simulink model "mpc_bike_model"  (R2018b)
settings: Solver=ode23s  StartTime=0.0  StopTime=sim_time  FixedStep=Ts_IMU  MaxStep=Ts  RelTol=1e-3
values from neighbouring files (symbols this model uses):
  A_kalman = [1 0 Ts 0; 0 1 0 Ts; 0 0 1 0; 0 0 0 1]    [configuration_boxMovedCenter.m]    (also in configuration_lqrTuning.m; configuration_pidTuning.m; configuration_yixiao.m)
  b_compFilter = b_real    (= 1.095)    [configuration_boxMovedCenter.m]    (also in configuration_lqrTuning.m; configuration_pidTuning.m; configuration_yixiao.m)
  B_kalman = [0 0 0 0; 0 0 0 0; 0 0 0 0; 0 0 0 0]    [configuration_boxMovedCenter.m]    (also in configuration_lqrTuning.m; configuration_pidTuning.m; configuration_yixiao.m)
  b_real = 1.095    [configuration_boxMovedCenter.m]    (also in configuration_lqrTuning.m; configuration_pidTuning.m; configuration_yixiao.m)
  C_kalman = [1 0 0 0; 0 1 0 0; 0 0 1 0; 0 0 0 1]    [configuration_boxMovedCenter.m]    (also in configuration_lqrTuning.m; configuration_pidTuning.m; configuration_yixiao.m)
  complementary = 0.985    [configuration_boxMovedCenter.m]    (also in configuration_lqrTuning.m; configuration_pidTuning.m; configuration_yixiao.m)
  D_kalman = [0 0 0 0; 0 0 0 0; 0 0 0 0; 0 0 0 0]    [configuration_boxMovedCenter.m]    (also in configuration_lqrTuning.m; configuration_pidTuning.m; configuration_yixiao.m)
  damp = 0.4    [configuration_boxMovedCenter.m]    (also in configuration_lqrTuning.m; configuration_pidTuning.m; configuration_yixiao.m)
  Dead_Band = [0.0, -0.0, 0.0]    [configuration_boxMovedCenter.m]    (also in configuration_lqrTuning.m = [0.055, -0.055, 0.005]; configuration_pidTuning.m = [0.055, -0.055, 0.005]; configuration_yixiao.m = [0.055, -0.055, 0.005])
  delay = 0.045    [configuration_boxMovedCenter.m]    (also in configuration_lqrTuning.m; configuration_pidTuning.m; configuration_yixiao.m)
  direct_control = 1    [configuration_boxMovedCenter.m]    (also in configuration_lqrTuning.m; configuration_pidTuning.m; configuration_yixiao.m)
  filter_model = 1    [configuration_boxMovedCenter.m]    (also in configuration_lqrTuning.m; configuration_pidTuning.m; configuration_yixiao.m)
  forward_motor_dynamics = 0    [configuration_boxMovedCenter.m]    (also in configuration_lqrTuning.m; configuration_pidTuning.m; configuration_yixiao.m)
  fr_oscil = 1    [configuration_boxMovedCenter.m]    (also in configuration_lqrTuning.m; configuration_pidTuning.m; configuration_yixiao.m)
  g = 9.81    [configuration_boxMovedCenter.m]    (also in configuration_lqrTuning.m; configuration_pidTuning.m; configuration_yixiao.m)
  gain = 0.3    [configuration_boxMovedCenter.m]    (also in configuration_lqrTuning.m; configuration_pidTuning.m; configuration_yixiao.m)
  I_direct = 0.4    [configuration_boxMovedCenter.m]    (also in configuration_lqrTuning.m = 0.000227125326188; configuration_pidTuning.m = 0.000227125326188; configuration_yixiao.m)
  I_lat = 0.01    [configuration_boxMovedCenter.m]    (also in configuration_lqrTuning.m = 0.000115580509654; configuration_pidTuning.m = 0.000115580509654; configuration_yixiao.m)
  I_steer = 0.1    [configuration_boxMovedCenter.m]    (also in configuration_lqrTuning.m = 0.451012019539; configuration_pidTuning.m = 0.451012019539; configuration_yixiao.m = 0.3)
  IMU_height_model = 0.45    [configuration_boxMovedCenter.m]    (also in configuration_lqrTuning.m; configuration_pidTuning.m; configuration_yixiao.m)
  IMU_height_real = 0.45    [configuration_boxMovedCenter.m]    (also in configuration_lqrTuning.m; configuration_pidTuning.m; configuration_yixiao.m)
  initial_states = [deg2rad(5) deg2rad(-2) deg2rad(0)]    [configuration_boxMovedCenter.m]    (also in configuration_lqrTuning.m = [deg2rad(-2) deg2rad(0) deg2rad(0)]; configuration_pidTuning.m = [deg2rad(-2) deg2rad(0) deg2rad(0)]; configuration_yixiao.m = [deg2rad(-2) deg2rad(0) deg2rad(0)])
  input_velocity = 3    [configuration_boxMovedCenter.m]    (also in configuration_lqrTuning.m; configuration_pidTuning.m; configuration_yixiao.m)
  lambda_compFilter = deg2rad(70)    [configuration_boxMovedCenter.m]    (also in configuration_lqrTuning.m; configuration_pidTuning.m; configuration_yixiao.m)
  lambda_real = deg2rad(70)    [configuration_boxMovedCenter.m]    (also in configuration_lqrTuning.m; configuration_pidTuning.m; configuration_yixiao.m)
  lat_control = 1    [configuration_boxMovedCenter.m]    (also in configuration_lqrTuning.m; configuration_pidTuning.m; configuration_yixiao.m)
  look_ahead = 0    [configuration_boxMovedCenter.m]    (also in configuration_lqrTuning.m; configuration_pidTuning.m; configuration_yixiao.m)
  max_handlebar = 40*(pi/180)    (= 0.698131700798)    [configuration_boxMovedCenter.m]    (also in configuration_lqrTuning.m; configuration_pidTuning.m; configuration_yixiao.m)
  max_roll = pi/2    (= 1.57079632679)    [configuration_boxMovedCenter.m]    (also in configuration_lqrTuning.m; configuration_pidTuning.m; configuration_yixiao.m)
  max_steering_motor_acc = inf    [configuration_boxMovedCenter.m]    (also in configuration_lqrTuning.m; configuration_pidTuning.m; configuration_yixiao.m)
  max_steering_motor_speed = 7.5    [configuration_boxMovedCenter.m]    (also in configuration_lqrTuning.m; configuration_pidTuning.m; configuration_yixiao.m)
  min_handlebar = -max_handlebar    (= -0.698131700798)    [configuration_boxMovedCenter.m]    (also in configuration_lqrTuning.m; configuration_pidTuning.m; configuration_yixiao.m)
  min_roll = - max_roll    (= -1.57079632679)    [configuration_boxMovedCenter.m]    (also in configuration_lqrTuning.m; configuration_pidTuning.m; configuration_yixiao.m)
  min_steering_motor_acc = -inf    [configuration_boxMovedCenter.m]    (also in configuration_lqrTuning.m; configuration_pidTuning.m; configuration_yixiao.m)
  min_steering_motor_speed = -7.5    [configuration_boxMovedCenter.m]    (also in configuration_lqrTuning.m; configuration_pidTuning.m; configuration_yixiao.m)
  noise = 1    [configuration_boxMovedCenter.m]    (also in configuration_lqrTuning.m = 0; configuration_pidTuning.m = 0; configuration_yixiao.m = 0)
  noise_acc = 2.4869e-05    [configuration_boxMovedCenter.m]    (also in configuration_lqrTuning.m; configuration_pidTuning.m; configuration_yixiao.m)
  noise_encoder = 1e-7    (= 1e-07)    [configuration_boxMovedCenter.m]    (also in configuration_lqrTuning.m; configuration_pidTuning.m; configuration_yixiao.m)
  noise_gyro = 0.0022    [configuration_boxMovedCenter.m]    (also in configuration_lqrTuning.m; configuration_pidTuning.m; configuration_yixiao.m)
  noise_hall = 0.0031    [configuration_boxMovedCenter.m]    (also in configuration_lqrTuning.m; configuration_pidTuning.m; configuration_yixiao.m)
  noise_pos_meas = 0.51    [configuration_boxMovedCenter.m]    (also in configuration_lqrTuning.m; configuration_pidTuning.m; configuration_yixiao.m)
  osc_roll = 0    [configuration_boxMovedCenter.m]    (also in configuration_lqrTuning.m; configuration_pidTuning.m; configuration_yixiao.m)
  osc_steer = 0    [configuration_boxMovedCenter.m]    (also in configuration_lqrTuning.m; configuration_pidTuning.m; configuration_yixiao.m)
  P_direct = 0.8    [configuration_boxMovedCenter.m]    (also in configuration_lqrTuning.m = 0.0712859744207; configuration_pidTuning.m = 0.0712859744207; configuration_yixiao.m)
  P_lat = 0.1    [configuration_boxMovedCenter.m]    (also in configuration_lqrTuning.m = 0.0465435246389; configuration_pidTuning.m = 0.0465435246389; configuration_yixiao.m)
  P_steer = 1    [configuration_boxMovedCenter.m]    (also in configuration_lqrTuning.m = 0.219020351849; configuration_pidTuning.m = 0.219020351849; configuration_yixiao.m = 0.4)
  parameters_compFilter = [g h_compFilter b_compFilter a_compFilter lambda_compFilter c_compFilter]    [configuration_boxMovedCenter.m]    (also in configuration_lqrTuning.m; configuration_pidTuning.m; configuration_yixiao.m)
  parameters_f_b_real = [m_frame_real m_box_real h_frame_real h_box_real a_frame_real a_box_real c_frame_real c_box_real b_frame_real b_box_real l_frame_real l_box_real]    [configuration_boxMovedCenter.m]    (also in configuration_lqrTuning.m; configuration_pidTuning.m; configuration_yixiao.m = [m_frame_real m_box_real h_frame_real h_box_real a_frame_rea)
  parameters_real = [g h_real b_real a_real lambda_real c_real]    [configuration_boxMovedCenter.m]    (also in configuration_lqrTuning.m; configuration_pidTuning.m; configuration_yixiao.m)
  path_tracking = 0    [configuration_boxMovedCenter.m]    (also in configuration_lqrTuning.m = 1; configuration_pidTuning.m = 1; configuration_yixiao.m)
  plant_model = 1    [configuration_boxMovedCenter.m]    (also in configuration_lqrTuning.m; configuration_pidTuning.m; configuration_yixiao.m)
  R_kalman = [noise_pos_meas 0 0 0; 0 noise_pos_meas 0 0; 0 0 noise_hall 0; 0 0 0 noise_hall]    [configuration_boxMovedCenter.m]    (also in configuration_lqrTuning.m; configuration_pidTuning.m; configuration_yixiao.m)
  roll_rate_coef = 0.9    [configuration_boxMovedCenter.m]    (also in configuration_lqrTuning.m; configuration_pidTuning.m; configuration_yixiao.m)
  steer_control = 1    [configuration_boxMovedCenter.m]    (also in configuration_lqrTuning.m; configuration_pidTuning.m; configuration_yixiao.m)
  steering_motor_limitations = 1    [configuration_boxMovedCenter.m]    (also in configuration_lqrTuning.m; configuration_pidTuning.m; configuration_yixiao.m)
  Ts = 0.04    [configuration_boxMovedCenter.m]    (also in configuration_lqrTuning.m; configuration_pidTuning.m; configuration_yixiao.m)
  Ts_IMU = 0.04    [configuration_boxMovedCenter.m]    (also in configuration_lqrTuning.m; configuration_pidTuning.m; configuration_yixiao.m)
undefined symbols (not defined in the file or in its folder): A, B, cumulative_dist_along_path, curvature, DiscIntNeverNeededParam, Discrete, initial_x, initial_y, lqr_gains, path_x, path_y, sys_con, sys_dis, Time, velocity_lqr
libraries: simulink x14, simulink_extras x3, dspsigops x2, mpclib x1, ctrlSharedLib x1
(part 1 of 2)
settings Model: Creator=Boaz Ash  LastModifiedBy=maximef
settings DebuggingCC: UnconnectedInputMsg=none  UnconnectedOutputMsg=none  UnconnectedLineMsg=none  LibraryContextMissingDiagnostic=none
settings SFSimCC: SimUseLocalCustomCode=off
settings RTWCC: RTWUseLocalCustomCode=off

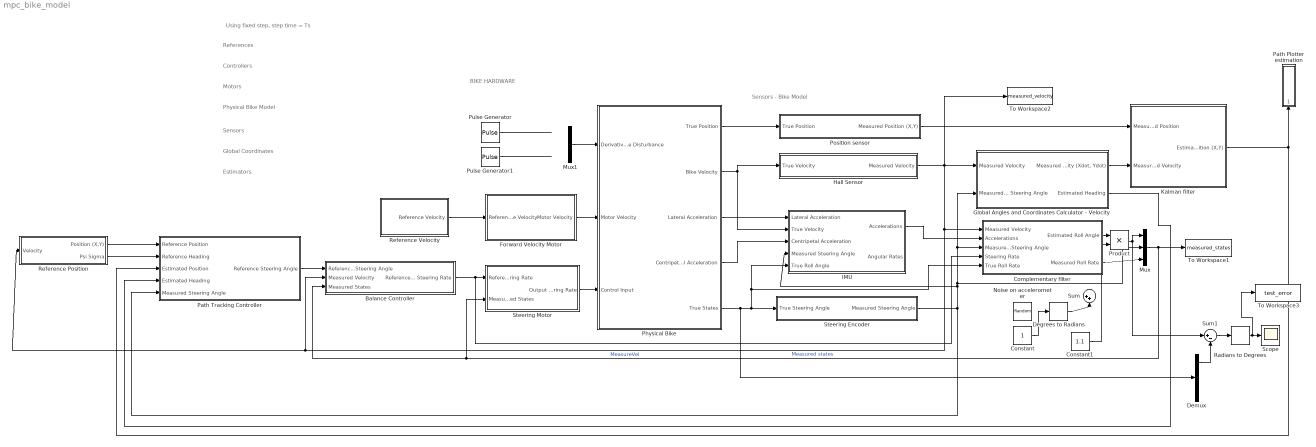
== system mpc_bike_model ==
  note: Using fixed step, step time = Ts
  note: BIKE HARDWARE
  note: References
  note: Physical Bike
      | Model
  note: Sensors - Bike Model
  note: Motors
  note: Sensors
  note: Global Coordinates
  note: Controllers
  note: Estimators
  Balance Controller : Subsystem  TreatAsAtomicUnit=on  SystemSampleTime=Ts
  Complementary filter : Subsystem  SystemSampleTime=Ts_IMU
  Constant : Constant
  Constant1 : Constant  Value=1.1
  Degrees to Radians : simulink_extras/Transformations/Degrees to Radians
  Demux : Demux  Outputs=3
  Forward Velocity Motor : Subsystem
  Global Angles and Coordinates Calculator - Velocity : Subsystem  SystemSampleTime=Ts
  Hall Sensor : Subsystem  TreatAsAtomicUnit=on  SystemSampleTime=Ts
  IMU : Subsystem  TreatAsAtomicUnit=on
  "Kalman filter " : Subsystem  SystemSampleTime=Ts
  Mux : Mux  Inputs=3
  Mux1 : Mux  Inputs=3
  Noise on accelerometer : RandomNumber  Variance=noise_acc  SampleTime=Ts
  Path Plotter estimation : Subsystem  SystemSampleTime=Ts
  Path Tracking Controller : Subsystem
  Physical Bike : Subsystem
  Position sensor : Subsystem  TreatAsAtomicUnit=on  SystemSampleTime=Ts
  Product : Product
  Pulse Generator : DiscretePulseGenerator  PulseType=Time based  Amplitude=pi/36  Period=100  PhaseDelay=1
  Pulse Generator1 : DiscretePulseGenerator  PulseType=Time based  Amplitude=-deg2rad(30)  Period=10  PulseWidth=10  PhaseDelay=1
  Radians to Degrees : simulink_extras/Transformations/Radians to Degrees
  "Reference Position " : Subsystem
  "Reference Velocity " : Subsystem
  Scope : Scope
  Steering Encoder : Subsystem  TreatAsAtomicUnit=on  SystemSampleTime=Ts
  Steering Motor : Subsystem
  Sum : Sum  Inputs=|++
  Sum1 : Sum  Inputs=|+-
  To Workspace1 : ToWorkspace  VariableName=measured_states  SaveFormat=Timeseries  SampleTime=-1
  To Workspace2 : ToWorkspace  VariableName=measured_velocity  SaveFormat=Timeseries  SampleTime=-1
  To Workspace3 : ToWorkspace  VariableName=test_error  SaveFormat=Structure With Time  SampleTime=-1
      settings: Save2DSignal=2-D array (concatenate along first dimension)
  wires:
  Mux1/1 -> Physical Bike/1(Derivative Disturbance)
  "Reference Velocity "/1(Reference Velocity) -> Forward Velocity Motor/1(Reference Velocity)
  Forward Velocity Motor/1(Motor Velocity) -> Physical Bike/2(Motor Velocity)
  Pulse Generator/1 -> ?
  Pulse Generator1/1 -> ?
  "Kalman filter "/1(Estimated Position (X,Y)) -> Path Tracking Controller/3(Estimated Position), Path Plotter estimation/1(Position)
  Global Angles and Coordinates Calculator - Velocity/2(Estimated Heading) -> Path Tracking Controller/4(Estimated Heading)
  Path Tracking Controller/1(Reference Steering Angle) -> Balance Controller/1(Reference Steering Angle)
  Balance Controller/1(Reference Steering Rate) -> Complementary filter/4(Steering Rate), Steering Motor/1(Reference Steering Rate)
  Physical Bike/3(Lateral Acceleration) -> IMU/1(Lateral Acceleration)
  Physical Bike/4(Centripetal Acceleration) -> IMU/3(Centripetal Acceleration)
  Mux/1 -> Steering Motor/2(Measured States), Balance Controller/3(Measured States), To Workspace1/1  "Measured states"
  Steering Motor/1(Output Steering Rate) -> Physical Bike/3(Control Input)
  Steering Encoder/1(Measured Steering Angle) -> Mux/2, Global Angles and Coordinates Calculator - Velocity/2("Measured Steering Angle "), Complementary filter/3(Measured Steering Angle), IMU/4(Measured Steering Angle), Path Tracking Controller/5(Measured Steering Angle)
  IMU/1(Accelerations) -> Complementary filter/2(Accelerations)
  Position sensor/1("Measured Position (X,Y) ") -> "Kalman filter "/1("Measured Position ")
  Physical Bike/1(True Position) -> Position sensor/1(True Position)
  Global Angles and Coordinates Calculator - Velocity/1("Measured Velocity (Xdot, Ydot)") -> "Kalman filter "/2(Measured Velocity)
  Complementary filter/2(Measured Roll Rate) -> Mux/3
  Hall Sensor/1(Measured Velocity) -> To Workspace2/1, Complementary filter/1(Measured Velocity), "Reference Position "/1(Velocity), Balance Controller/2(Measured Velocity), Global Angles and Coordinates Calculator - Velocity/1(Measured Velocity)  "MeasureVel"
  "Reference Position "/2(Psi Sigma) -> Path Tracking Controller/2(Reference Heading)
  "Reference Position "/1(Position (X,Y)) -> Path Tracking Controller/1(Reference Position)
  Physical Bike/5(True States) -> Demux/1, Complementary filter/5(True Roll Rate), IMU/5(True Roll Angle), Steering Encoder/1(True Steering Angle)
  Physical Bike/2(Bike Velocity) -> IMU/2(True Velocity), Hall Sensor/1(True Velocity)
  Complementary filter/1(Estimated Roll Angle) -> Product/1
  Product/1 -> Mux/1, Sum1/1
  Constant/1 -> Degrees to Radians/1
  Sum1/1 -> Radians to Degrees/1
  Demux/1 -> Sum1/2
  Degrees to Radians/1 -> Sum/2
  Constant1/1 -> Product/2
  Radians to Degrees/1 -> To Workspace3/1, Scope/1

== system mpc_bike_model/Balance Controller ==
  Reference Steering Angle : Inport
  Measured Velocity : Inport  Port=2
  Measured States : Inport  Port=3
  Delay : Delay  DelayLength=1  InitialCondition=[0;0;0]
  Delay1 : Delay  DelayLength=1  InitialCondition=[0;0;0]
  LQR Controller : Subsystem  Commented=on  TreatAsAtomicUnit=on  SystemSampleTime=Ts
  MPC Controller : mpclib/MPC Controller  SCDEnableBlockLinearizationSpecification=on  mpcobj=K_dis  is_multiple=0  enable_value=0  return_u0=off  updateMPCinCallerWorkspace=on  md_inport=off  mv_inport=off  return_cost=off  return_mvseq=off  return_qpstatus=off  return_xseq=off  return_state=off  return_ovseq=off  state_inport=off  umin_inport=off  umax_inport=off  ymin_inport=off  ymax_inport=off  cc_inport=off  ywt_inport=off  uwt_inport=off  duwt_inport=off  rhoeps_inport=off  uref_inport=off  n_ts=0.04  n_p=10  n_mv=1  n_md=0  n_ud=0  n_mo=3  n_uo=0  BlockDataType=double  SampleTimeInherited=off  switch_inport=off
  Reference States : Subsystem  SystemSampleTime=Ts
  Sum : Sum  Inputs=|+-
  To Workspace : ToWorkspace  VariableName=states_measured  SaveFormat=Timeseries  SampleTime=-1
  Reference Steering Rate : Outport
  wires:
  Reference States/1(Reference States) -> Sum/1, Delay1/1
  Sum/1 -> LQR Controller/2(State Error)
  MPC Controller/1 -> Reference Steering Rate/1
  Reference Steering Angle/1 -> Reference States/2(Delta Ref)
  Measured Velocity/1 -> Reference States/1(Velocity), LQR Controller/1(Velocity)
  Measured States/1 -> To Workspace/1, Sum/2, Delay/1
  Delay/1 -> MPC Controller/1
  Delay1/1 -> MPC Controller/2

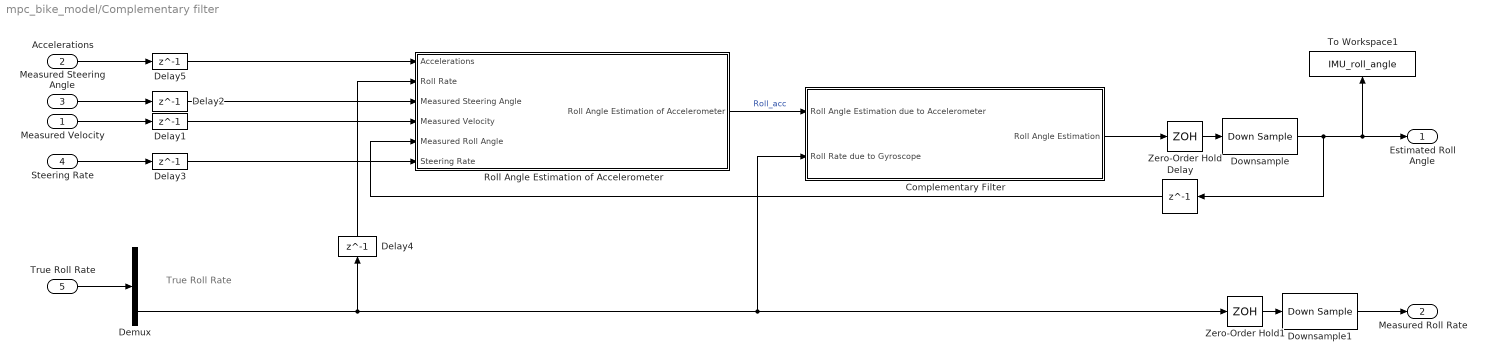
== system mpc_bike_model/Complementary filter ==
  note: True Roll
      | Rate
  Measured Velocity : Inport
  Accelerations : Inport  Port=2
  Measured Steering Angle : Inport  Port=3
  Steering Rate : Inport  Port=4
  True Roll Rate : Inport  Port=5
  Complementary Filter : Subsystem  TreatAsAtomicUnit=on  SystemSampleTime=Ts_IMU
  Delay{,1..2,4..5} (5 alike) : Delay  DelayLength=1
  Delay3 : Delay  DelayLength=1  SampleTime=Ts_IMU
  Demux : Demux  Outputs=3
  Downsample : DownSample  N=Ts/Ts_IMU  RateOptions=Allow multirate processing
  Downsample1 : DownSample  N=Ts/Ts_IMU  RateOptions=Allow multirate processing
  Roll Angle Estimation of Accelerometer : Subsystem
  To Workspace1 : ToWorkspace  VariableName=IMU_roll_angle  SaveFormat=Structure  SampleTime=-1
  Zero-Order Hold : ZeroOrderHold  SampleTime=Ts_IMU
  Zero-Order Hold1 : ZeroOrderHold  SampleTime=Ts_IMU
  Estimated Roll Angle : Outport
  Measured Roll Rate : Outport  Port=2
  wires:
  Roll Angle Estimation of Accelerometer/1(Roll Angle Estimation of Accelerometer) -> Complementary Filter/1(Roll Angle Estimation due to Accelerometer)  "Roll_acc"
  Demux/3 -> Zero-Order Hold1/1, Complementary Filter/2(Roll Rate due to Gyroscope), Delay4/1
  Zero-Order Hold/1 -> Downsample/1
  Zero-Order Hold1/1 -> Downsample1/1
  Accelerations/1 -> Delay5/1
  Measured Steering Angle/1 -> Delay2/1
  Measured Velocity/1 -> Delay1/1
  Delay/1 -> Roll Angle Estimation of Accelerometer/5(Measured Roll Angle)
  Delay1/1 -> Roll Angle Estimation of Accelerometer/4(Measured Velocity)
  Delay2/1 -> Roll Angle Estimation of Accelerometer/3(Measured Steering Angle)
  Steering Rate/1 -> Delay3/1
  Delay3/1 -> Roll Angle Estimation of Accelerometer/6(Steering Rate)
  Delay4/1 -> Roll Angle Estimation of Accelerometer/2(Roll Rate)
  Delay5/1 -> Roll Angle Estimation of Accelerometer/1(Accelerations)
  Complementary Filter/1(Roll Angle Estimation) -> Zero-Order Hold/1
  Downsample1/1 -> Measured Roll Rate/1
  Downsample/1 -> Estimated Roll Angle/1, To Workspace1/1, Delay/1
  True Roll Rate/1 -> Demux/1

== system mpc_bike_model/Forward Velocity Motor ==
  note: Add limit for acceleration/deceleration
      | Add min speed of 1.69 m/s (3600 rpm motor speed) limitation
      | Add min speed of 8.20 m/s (18000 rpm motor speed) limitation
      | Add deadband and delay
  Reference Velocity : Inport
  Band-Limited White Noise : simulink/Sources/Band-Limited White Noise  Cov=[0.001]  Ts=Ts  seed=[23341]
  Constant : Constant  Value=forward_motor_dynamics
  Rate Limiter : RateLimiter  RisingSlewLimit=inf  FallingSlewLimit=-inf  SampleTimeMode=inherited
  Saturation : Saturate  UpperLimit=inf  LowerLimit=0
  Sum : Sum  Inputs=|++
  Switch : Switch  Criteria=u2 > Threshold
  Transfer Fcn : TransferFcn  Numerator=[-0.2156 0.556]  Denominator=[1 1.675 0.5558]
  Motor Velocity : Outport
  wires:
  Reference Velocity/1 -> Transfer Fcn/1, Switch/3
  Transfer Fcn/1 -> Rate Limiter/1
  Switch/1 -> Sum/1
  Constant/1 -> Switch/2
  Saturation/1 -> Switch/1
  Rate Limiter/1 -> Saturation/1
  Sum/1 -> Motor Velocity/1

== system mpc_bike_model/Global Angles and Coordinates Calculator - Velocity ==
  Measured Velocity : Inport
  "Measured Steering Angle " : Inport  Port=2
  Discrete-Time Integrator : DiscreteIntegrator  SampleTime=-1  ICPrevOutput=DiscIntNeverNeededParam  ICPrevScaledInput=DiscIntNeverNeededParam
  Gain1 : Gain  Gain=sin(lambda_compFilter)
  Measured Bike Angles to Global Angles : Subsystem
  Measured Global Angles to Global Coordinates : Subsystem
  Sum : Sum  Inputs=++|
  To Workspace1 : ToWorkspace  VariableName=pos_vel_int  SaveFormat=Timeseries  SampleTime=-1
  "Measured Velocity (Xdot, Ydot)" : Outport
  Estimated Heading : Outport  Port=2
  wires:
  "Measured Steering Angle "/1 -> Gain1/1
  Measured Bike Angles to Global Angles/1(Psi) -> Sum/2, Measured Global Angles to Global Coordinates/2(Psi)
  Gain1/1 -> Measured Bike Angles to Global Angles/2(Measured Steering Angle)
  Sum/1 -> Estimated Heading/1
  Measured Bike Angles to Global Angles/2(Beta) -> Measured Global Angles to Global Coordinates/3(Beta), Sum/1
  Measured Velocity/1 -> Measured Bike Angles to Global Angles/1(Velocity), Measured Global Angles to Global Coordinates/1(Velocity)
  Measured Global Angles to Global Coordinates/1("Velocity (Xdot, Ydot)") -> "Measured Velocity (Xdot, Ydot)"/1, Discrete-Time Integrator/1
  Discrete-Time Integrator/1 -> To Workspace1/1

== system mpc_bike_model/Hall Sensor ==
  note: Switch Noise
  True Velocity : Inport
  Gain1 : Gain  Gain=noise
  Gain2 : Gain  Gain=1-noise
  Noise on hall sensor : RandomNumber  Variance=noise_hall  SampleTime=Ts
  Saturate Signal : Switch  Criteria=u2 > Threshold
  Sum : Sum  Inputs=++|
  Sum1 : Sum  Inputs=|++
  To Workspace3 : ToWorkspace  VariableName=vel_meas  SaveFormat=Timeseries  SampleTime=-1
  Velocity Lower Bound : simulink/Model Verification/Check Static  Lower Bound  Description=0.6 <= u  min=0.6  min_included=on  enabled=on  stopWhenAssertionFail=off  export=on  icon=graphic
      settings: SourceProductName=Simulink
  Zero : Constant  Value=0
  Zero-Order Hold : ZeroOrderHold  SampleTime=Ts
  Measured Velocity : Outport
  wires:
  Sum1/1 -> Saturate Signal/1, Velocity Lower Bound/1
  Noise on hall sensor/1 -> Sum/1
  Zero/1 -> Saturate Signal/3
  Velocity Lower Bound/1 -> Saturate Signal/2
  Saturate Signal/1 -> Zero-Order Hold/1
  Zero-Order Hold/1 -> Measured Velocity/1, To Workspace3/1
  True Velocity/1 -> Gain2/1, Sum/2
  Gain1/1 -> Sum1/1
  Gain2/1 -> Sum1/2
  Sum/1 -> Gain1/1

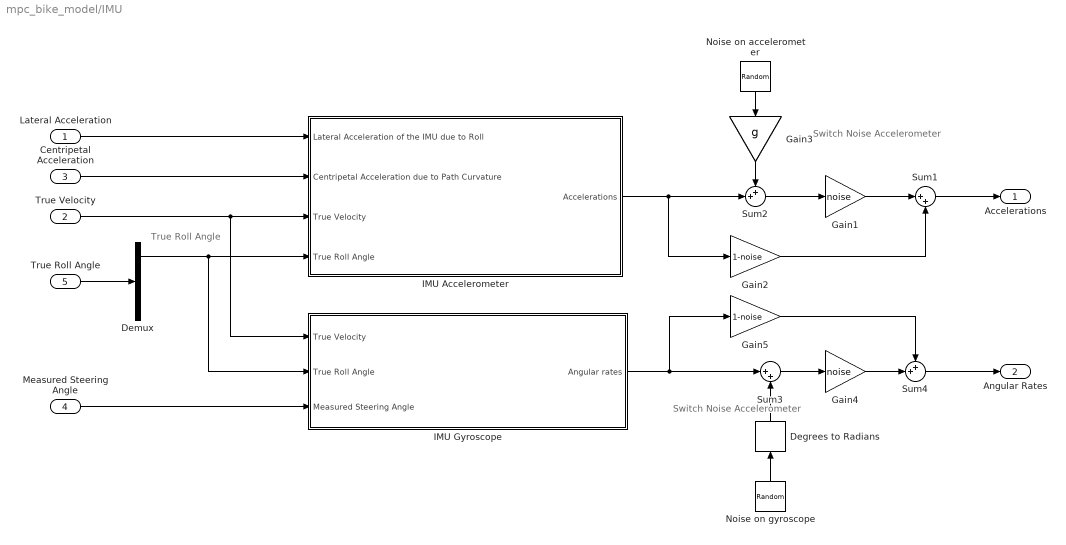
== system mpc_bike_model/IMU ==
  note: True Roll
      | Angle
  note: Switch Noise
      | Accelerometer
  note: Switch Noise
      | Accelerometer
  Lateral Acceleration : Inport
  True Velocity : Inport  Port=2
  Centripetal Acceleration : Inport  Port=3
  Measured Steering Angle : Inport  Port=4
  True Roll Angle : Inport  Port=5
  Degrees to Radians : simulink_extras/Transformations/Degrees to Radians
  Demux : Demux  Outputs=3
  Gain1 : Gain  Gain=noise
  Gain2 : Gain  Gain=1-noise
  Gain3 : Gain  Gain=g
  Gain4 : Gain  Gain=noise
  Gain5 : Gain  Gain=1-noise
  IMU Accelerometer : Subsystem
  IMU Gyroscope : Subsystem
  Noise on accelerometer : RandomNumber  Variance=noise_acc  SampleTime=Ts
  Noise on gyroscope : RandomNumber  Variance=noise_gyro  SampleTime=Ts
  Sum1 : Sum  Inputs=|++
  Sum2 : Sum  Inputs=++|
  Sum3 : Sum  Inputs=|++
  Sum4 : Sum  Inputs=++|
  Accelerations : Outport
  Angular Rates : Outport  Port=2
  wires:
  Measured Steering Angle/1 -> IMU Gyroscope/3(Measured Steering Angle)
  True Velocity/1 -> IMU Gyroscope/1(True Velocity), IMU Accelerometer/3(True Velocity)
  Lateral Acceleration/1 -> IMU Accelerometer/1(Lateral Acceleration of the IMU due to Roll)
  Centripetal Acceleration/1 -> IMU Accelerometer/2(Centripetal Acceleration due to Path Curvature)
  True Roll Angle/1 -> Demux/1
  Demux/1 -> IMU Gyroscope/2(True Roll Angle), IMU Accelerometer/4(True Roll Angle)
  Gain2/1 -> Sum1/2
  Sum1/1 -> Accelerations/1
  IMU Accelerometer/1(Accelerations) -> Sum2/2, Gain2/1
  Noise on accelerometer/1 -> Gain3/1
  Gain3/1 -> Sum2/1
  Noise on gyroscope/1 -> Degrees to Radians/1
  IMU Gyroscope/1(Angular rates) -> Sum3/1, Gain5/1
  Degrees to Radians/1 -> Sum3/2
  Gain5/1 -> Sum4/1
  Sum4/1 -> Angular Rates/1
  Sum3/1 -> Gain4/1
  Gain4/1 -> Sum4/2
  Sum2/1 -> Gain1/1
  Gain1/1 -> Sum1/1

== system mpc_bike_model/Kalman filter  ==
  note: y_k
  note: Measurements
  "Measured Position " : Inport
  Measured Velocity : Inport  Port=2
  Demux : Demux  Outputs=2
  "Kalman Filter " : ctrlSharedLib/Kalman Filter  TimeDomain=Discrete-Time  UseCurrentEstimator=on  ModelSource=Individual A, B, C, D matrices  ModelSourceVariable=ss(0.95,1,1,0,1)  A=A_kalman  B=B_kalman  C=C_kalman  D=D_kalman  NumberOfStates=1  NumberOfInputs=1  NumberOfOutputs=1  InitialEstimateSource=Dialog  X0=0  P0=10  UseK=off  UseGH=off  NumberOfProcessNoiseInputs=1  G=1  TimeInvariantG=on  H=0  TimeInvariantH=on  Q=Q_kalman  TimeInvariantQ=on  R=R_kalman  TimeInvariantR=on  N=0  TimeInvariantN=on  AddInputPort=on  AddEnablePort=off  OutputEstimatedY=off  OutputP=off  Ts=Ts
      settings: SourceProductBaseCode=CT
  Mux : Mux  Inputs=2
  Zero-Order Hold : ZeroOrderHold  SampleTime=-1
  Estimated Position (X,Y) : Outport
  wires:
  Measured Velocity/1 -> Mux/2
  Mux/1 -> Zero-Order Hold/1
  "Measured Position "/1 -> Mux/1
  "Kalman Filter "/1 -> Demux/1
  Demux/1 -> Estimated Position (X,Y)/1
  Zero-Order Hold/1 -> "Kalman Filter "/2

== system mpc_bike_model/Path Plotter estimation ==
  Position : Inport
  Demux : Demux  Outputs=2
  To Workspace : ToWorkspace  VariableName=X_BIKE_estim  SaveFormat=Timeseries  SampleTime=Ts
  To Workspace1 : ToWorkspace  VariableName=Y_BIKE_estim  SaveFormat=Timeseries  SampleTime=Ts
  XY Graph : simulink/Sinks/XY Graph  Commented=on  xmin=min(path_x)-5  xmax=max(path_x)+5  ymin=min(path_y)-5  ymax=max(path_y)+5  st=-1
  wires:
  Demux/1 -> XY Graph/1, To Workspace/1  "X"
  Demux/2 -> XY Graph/2, To Workspace1/1  "Y"
  Position/1 -> Demux/1

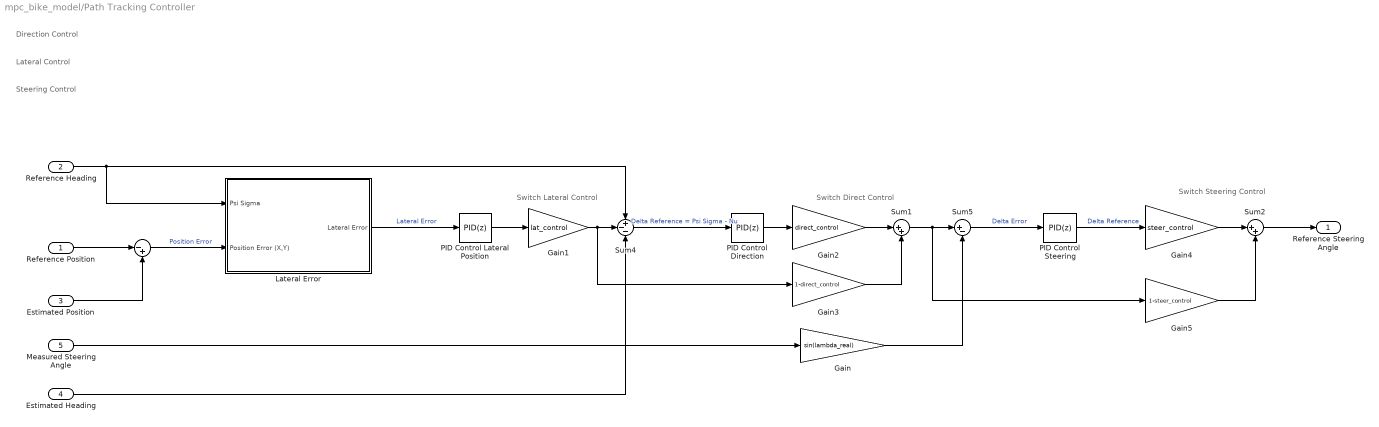
== system mpc_bike_model/Path Tracking Controller ==
  note: Switch Steering Control
  note: Direction Control
  note: Lateral Control
  note: Steering Control
  note: Switch Direct Control
  note: Switch Lateral Control
  Reference Position : Inport
  Reference Heading : Inport  Port=2
  Estimated Position : Inport  Port=3
  Estimated Heading : Inport  Port=4
  Measured Steering Angle : Inport  Port=5
  " " : Sum  Inputs=|-+
  Gain : Gain  Gain=sin(lambda_real)
  Gain1 : Gain  Gain=lat_control
  Gain2 : Gain  Gain=direct_control
  Gain3 : Gain  Gain=1-direct_control
  Gain4 : Gain  Gain=steer_control
  Gain5 : Gain  Gain=1-steer_control
  Lateral Error : Subsystem  SystemSampleTime=Ts
  PID Control Lateral Position : simulink/Continuous/PID Controller  Controller=PID  Form=Parallel  TimeDomain=Discrete-time  SampleTime=Ts  IntegratorMethod=Forward Euler  FilterMethod=Forward Euler  ControllerParametersSource=internal  P=P_lat  I=I_lat  D=0  UseFilter=on  N=100  TunerSelectOption=Transfer Function Based (PID Tuner App)  InitialConditionSource=internal  InitialConditionForIntegrator=0  InitialConditionForFilter=0  DifferentiatorICPrevScaledInput=0  ExternalReset=none  TrackingMode=off  Kt=1  LimitOutput=off  UpperSaturationLimit=inf  LowerSaturationLimit=-inf  LinearizeAsGain=on  AntiWindupMode=none  Kb=1  POutMin=[]  POutMax=[]  IOutMin=[]  IOutMax=[]  DOutMin=[]  DOutMax=[]  NOutMin=[]  NOutMax=[]  SumOutMin=[]  SumOutMax=[]  SaturationOutMin=[]  SaturationOutMax=[]  PParamMin=[]  PParamMax=[]  IParamMin=[]  IParamMax=[]  DParamMin=[]  DParamMax=[]  NParamMin=[]  NParamMax=[]  KbParamMin=[]  KbParamMax=[]  KtParamMin=[]  KtParamMax=[]  KbOutMin=[]  KbOutMax=[]  KtOutMin=[]  KtOutMax=[]  IntegratorOutMin=[]  IntegratorOutMax=[]  FilterOutMin=[]  FilterOutMax=[]  SumI1OutMin=[]  SumI1OutMax=[]  SumI2OutMin=[]  SumI2OutMax=[]  SumI3OutMin=[]  SumI3OutMax=[]  SumI4OutMin=[]  SumI4OutMax=[]  SumDOutMin=[]  SumDOutMax=[]  DifferentiatorOutMin=[]  DifferentiatorOutMax=[]  FilterDiffOutCoefMin=[]  FilterDiffOutCoefMax=[]  ReciprocalOutMin=[]  ReciprocalOutMax=[]  SumDenOutMin=[]  SumDenOutMax=[]  SumNumOutMin=[]  SumNumOutMax=[]  DivideOutMin=[]  DivideOutMax=[]  IntegratorContinuousStateAttributes=''  IntegratorStateMustResolveToSignalObject=off  IntegratorRTWStateStorageClass=Auto  FilterContinuousStateAttributes=''  FilterStateMustResolveToSignalObject=off  FilterRTWStateStorageClass=Auto  ParallelPVariant=InternalParameters  IdealPVariant=Disabled  IVariant=InternalParameters  DVariant=InternalParameters  IntegratorVariant=Discrete  SatVariant=Disabled  AWVariant=Passthrough  PCopyVariant=Disabled  TRVariant=Disabled  FdbkBlocksVariant=Forward  IdealPFdbkVariant=Disabled  SatFdbkVariant=Disabled  DerivativeFilterVariant=ForwardEulerFilter  NVariant=InternalParameters  NCopyVariant=Disabled  FilterICVariant=InternalICsFilter  IntegratorICVariant=InternalICs  ExternalResetVariant=Disabled  TRSumVariant=Passthrough  SumFdbkVariant=Disabled  SumVariant=Sum_PID
  PID Control Direction : simulink/Continuous/PID Controller  Controller=PID  Form=Parallel  TimeDomain=Discrete-time  SampleTime=Ts  IntegratorMethod=Forward Euler  FilterMethod=Forward Euler  ControllerParametersSource=internal  P=P_direct  I=I_direct  D=0  UseFilter=on  N=100  TunerSelectOption=Transfer Function Based (PID Tuner App)  InitialConditionSource=internal  InitialConditionForIntegrator=0  InitialConditionForFilter=0  DifferentiatorICPrevScaledInput=0  ExternalReset=none  TrackingMode=off  Kt=1  LimitOutput=off  UpperSaturationLimit=inf  LowerSaturationLimit=-inf  LinearizeAsGain=on  AntiWindupMode=none  Kb=1  POutMin=[]  POutMax=[]  IOutMin=[]  IOutMax=[]  DOutMin=[]  DOutMax=[]  NOutMin=[]  NOutMax=[]  SumOutMin=[]  SumOutMax=[]  SaturationOutMin=[]  SaturationOutMax=[]  PParamMin=[]  PParamMax=[]  IParamMin=[]  IParamMax=[]  DParamMin=[]  DParamMax=[]  NParamMin=[]  NParamMax=[]  KbParamMin=[]  KbParamMax=[]  KtParamMin=[]  KtParamMax=[]  KbOutMin=[]  KbOutMax=[]  KtOutMin=[]  KtOutMax=[]  IntegratorOutMin=[]  IntegratorOutMax=[]  FilterOutMin=[]  FilterOutMax=[]  SumI1OutMin=[]  SumI1OutMax=[]  SumI2OutMin=[]  SumI2OutMax=[]  SumI3OutMin=[]  SumI3OutMax=[]  SumI4OutMin=[]  SumI4OutMax=[]  SumDOutMin=[]  SumDOutMax=[]  DifferentiatorOutMin=[]  DifferentiatorOutMax=[]  FilterDiffOutCoefMin=[]  FilterDiffOutCoefMax=[]  ReciprocalOutMin=[]  ReciprocalOutMax=[]  SumDenOutMin=[]  SumDenOutMax=[]  SumNumOutMin=[]  SumNumOutMax=[]  DivideOutMin=[]  DivideOutMax=[]  IntegratorContinuousStateAttributes=''  IntegratorStateMustResolveToSignalObject=off  IntegratorRTWStateStorageClass=Auto  FilterContinuousStateAttributes=''  FilterStateMustResolveToSignalObject=off  FilterRTWStateStorageClass=Auto  ParallelPVariant=InternalParameters  IdealPVariant=Disabled  IVariant=InternalParameters  DVariant=InternalParameters  IntegratorVariant=Discrete  SatVariant=Disabled  AWVariant=Passthrough  PCopyVariant=Disabled  TRVariant=Disabled  FdbkBlocksVariant=Forward  IdealPFdbkVariant=Disabled  SatFdbkVariant=Disabled  DerivativeFilterVariant=ForwardEulerFilter  NVariant=InternalParameters  NCopyVariant=Disabled  FilterICVariant=InternalICsFilter  IntegratorICVariant=InternalICs  ExternalResetVariant=Disabled  TRSumVariant=Passthrough  SumFdbkVariant=Disabled  SumVariant=Sum_PID
  PID Control Steering : simulink/Continuous/PID Controller  Controller=PID  Form=Parallel  TimeDomain=Discrete-time  SampleTime=Ts  IntegratorMethod=Forward Euler  FilterMethod=Forward Euler  ControllerParametersSource=internal  P=P_steer  I=I_steer  D=0  UseFilter=on  N=100  TunerSelectOption=Transfer Function Based (PID Tuner App)  InitialConditionSource=internal  InitialConditionForIntegrator=0  InitialConditionForFilter=0  DifferentiatorICPrevScaledInput=0  ExternalReset=none  TrackingMode=off  Kt=1  LimitOutput=off  UpperSaturationLimit=inf  LowerSaturationLimit=-inf  LinearizeAsGain=on  AntiWindupMode=none  Kb=1  POutMin=[]  POutMax=[]  IOutMin=[]  IOutMax=[]  DOutMin=[]  DOutMax=[]  NOutMin=[]  NOutMax=[]  SumOutMin=[]  SumOutMax=[]  SaturationOutMin=[]  SaturationOutMax=[]  PParamMin=[]  PParamMax=[]  IParamMin=[]  IParamMax=[]  DParamMin=[]  DParamMax=[]  NParamMin=[]  NParamMax=[]  KbParamMin=[]  KbParamMax=[]  KtParamMin=[]  KtParamMax=[]  KbOutMin=[]  KbOutMax=[]  KtOutMin=[]  KtOutMax=[]  IntegratorOutMin=[]  IntegratorOutMax=[]  FilterOutMin=[]  FilterOutMax=[]  SumI1OutMin=[]  SumI1OutMax=[]  SumI2OutMin=[]  SumI2OutMax=[]  SumI3OutMin=[]  SumI3OutMax=[]  SumI4OutMin=[]  SumI4OutMax=[]  SumDOutMin=[]  SumDOutMax=[]  DifferentiatorOutMin=[]  DifferentiatorOutMax=[]  FilterDiffOutCoefMin=[]  FilterDiffOutCoefMax=[]  ReciprocalOutMin=[]  ReciprocalOutMax=[]  SumDenOutMin=[]  SumDenOutMax=[]  SumNumOutMin=[]  SumNumOutMax=[]  DivideOutMin=[]  DivideOutMax=[]  IntegratorContinuousStateAttributes=''  IntegratorStateMustResolveToSignalObject=off  IntegratorRTWStateStorageClass=Auto  FilterContinuousStateAttributes=''  FilterStateMustResolveToSignalObject=off  FilterRTWStateStorageClass=Auto  ParallelPVariant=InternalParameters  IdealPVariant=Disabled  IVariant=InternalParameters  DVariant=InternalParameters  IntegratorVariant=Discrete  SatVariant=Disabled  AWVariant=Passthrough  PCopyVariant=Disabled  TRVariant=Disabled  FdbkBlocksVariant=Forward  IdealPFdbkVariant=Disabled  SatFdbkVariant=Disabled  DerivativeFilterVariant=ForwardEulerFilter  NVariant=InternalParameters  NCopyVariant=Disabled  FilterICVariant=InternalICsFilter  IntegratorICVariant=InternalICs  ExternalResetVariant=Disabled  TRSumVariant=Passthrough  SumFdbkVariant=Disabled  SumVariant=Sum_PID
  Sum1 : Sum  Inputs=|++
  Sum2 : Sum  Inputs=|++
  Sum4 : Sum  Inputs=+--
  Sum5 : Sum  Inputs=|+-
  Reference Steering Angle : Outport
  wires:
  Lateral Error/1(Lateral Error) -> PID Control Lateral Position/1  "Lateral Error"
  Sum5/1 -> PID Control Steering/1  "Delta Error"
  Estimated Position/1 -> " "/2
  " "/1 -> Lateral Error/2(Position Error (X,Y))  "Position Error"
  Sum4/1 -> PID Control Direction/1  "Delta Reference = Psi Sigma - Nu"
  Measured Steering Angle/1 -> Gain/1
  Estimated Heading/1 -> Sum4/3
  Gain/1 -> Sum5/2
  Gain1/1 -> Gain3/1, Sum4/2
  PID Control Lateral Position/1 -> Gain1/1
  Sum1/1 -> Gain5/1, Sum5/1
  PID Control Steering/1 -> Gain4/1  "Delta Reference"
  Sum2/1 -> Reference Steering Angle/1
  Gain4/1 -> Sum2/1
  Reference Heading/1 -> Lateral Error/1(Psi Sigma), Sum4/1
  Reference Position/1 -> " "/1
  PID Control Direction/1 -> Gain2/1
  Gain2/1 -> Sum1/1
  Gain3/1 -> Sum1/2
  Gain5/1 -> Sum2/2

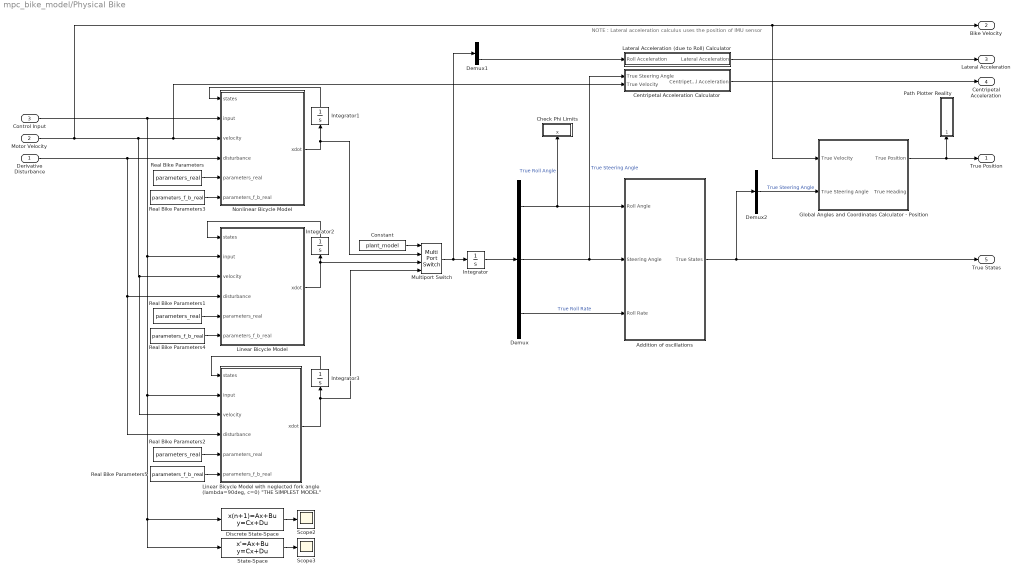
== system mpc_bike_model/Physical Bike ==
  note: NOTE : Lateral acceleration calculus uses the position of IMU sensor
  Derivative Disturbance : Inport
  Motor Velocity : Inport  Port=2
  Control Input : Inport  Port=3
  " Addition of oscillations" : Subsystem  SystemSampleTime=Ts
  Centripetal Acceleration Calculator : Subsystem
  Check Phi Limits : Subsystem  TreatAsAtomicUnit=on  SystemSampleTime=Ts
  Constant : Constant  Value=plant_model
  Demux : Demux  Outputs=3
  Demux1 : Demux  Outputs=3
  Demux2 : Demux  Outputs=3
  Discrete State-Space : DiscreteStateSpace  A=sys_dis.A  B=sys_dis.B  C=eye(3,3)  D=zeros(3,1)  SampleTime=Ts_IMU
  Global Angles and Coordinates Calculator - Position : Subsystem  SystemSampleTime=Ts
  Integrator{,1..3} (4 alike) : Integrator  InitialCondition=initial_states
  Lateral Acceleration (due to Roll) Calculator : Subsystem
  Linear Bicycle Model : MATLAB Function  TreatAsAtomicUnit=on
  "Linear Bicycle Model with neglected fork angle (lambda=90deg, c=0) \"THE SIMPLEST MODEL\"" : MATLAB Function  TreatAsAtomicUnit=on
  Multiport Switch : MultiPortSwitch
  Nonlinear Bicycle Model : MATLAB Function  TreatAsAtomicUnit=on
  Path Plotter Reality : Subsystem  SystemSampleTime=Ts
  Real Bike Parameters : Constant  Value=parameters_real
  Real Bike Parameters1 : Constant  Value=parameters_real
  Real Bike Parameters2 : Constant  Value=parameters_real
  Real Bike Parameters3 : Constant  Value=parameters_f_b_real
  Real Bike Parameters4 : Constant  Value=parameters_f_b_real
  Real Bike Parameters5 : Constant  Value=parameters_f_b_real
  Scope2 : Scope
  Scope3 : Scope
  State-Space : StateSpace  A=sys_con.A  B=sys_con.B  C=eye(3,3)  D=zeros(3,1)  InitialCondition=0
  True Position : Outport
  Bike Velocity : Outport  Port=2
  Lateral Acceleration : Outport  Port=3
  Centripetal Acceleration : Outport  Port=4
  True States : Outport  Port=5
  wires:
  Real Bike Parameters5/1 -> "Linear Bicycle Model with neglected fork angle (lambda=90deg, c=0) \"THE SIMPLEST MODEL\""/6(parameters_f_b_real)
  Demux/2 -> Centripetal Acceleration Calculator/1(True Steering Angle), " Addition of oscillations"/2(Steering Angle)  "True Steering Angle"
  Control Input/1 -> Nonlinear Bicycle Model/2(input), State-Space/1, Discrete State-Space/1, "Linear Bicycle Model with neglected fork angle (lambda=90deg, c=0) \"THE SIMPLEST MODEL\""/2(input), Linear Bicycle Model/2(input)
  Integrator1/1 -> Nonlinear Bicycle Model/1(states)
  Real Bike Parameters3/1 -> Nonlinear Bicycle Model/6(parameters_f_b_real)
  Constant/1 -> Multiport Switch/1
  Real Bike Parameters2/1 -> "Linear Bicycle Model with neglected fork angle (lambda=90deg, c=0) \"THE SIMPLEST MODEL\""/5(parameters_real)
  State-Space/1 -> Scope3/1
  Discrete State-Space/1 -> Scope2/1
  Integrator/1 -> Demux/1
  Demux/1 -> Check Phi Limits/1(x), " Addition of oscillations"/1(Roll Angle)  "True Roll Angle"
  Real Bike Parameters1/1 -> Linear Bicycle Model/5(parameters_real)
  Centripetal Acceleration Calculator/1(Centripetal Acceleration) -> Centripetal Acceleration/1
  Nonlinear Bicycle Model/1(xdot) -> Integrator1/1, Multiport Switch/2
  Demux1/3 -> Lateral Acceleration (due to Roll) Calculator/1(Roll Acceleration)
  Linear Bicycle Model/1(xdot) -> Integrator2/1, Multiport Switch/3
  Derivative Disturbance/1 -> "Linear Bicycle Model with neglected fork angle (lambda=90deg, c=0) \"THE SIMPLEST MODEL\""/4(disturbance), Linear Bicycle Model/4(disturbance), Nonlinear Bicycle Model/4(disturbance)
  Real Bike Parameters/1 -> Nonlinear Bicycle Model/5(parameters_real)
  "Linear Bicycle Model with neglected fork angle (lambda=90deg, c=0) \"THE SIMPLEST MODEL\""/1(xdot) -> Integrator3/1, Multiport Switch/4
  Multiport Switch/1 -> Demux1/1, Integrator/1
  Lateral Acceleration (due to Roll) Calculator/1(Lateral Acceleration) -> Lateral Acceleration/1
  Integrator3/1 -> "Linear Bicycle Model with neglected fork angle (lambda=90deg, c=0) \"THE SIMPLEST MODEL\""/1(states)
  Integrator2/1 -> Linear Bicycle Model/1(states)
  Motor Velocity/1 -> Global Angles and Coordinates Calculator - Position/1(True Velocity), Bike Velocity/1, Centripetal Acceleration Calculator/2(True Velocity), Nonlinear Bicycle Model/3(velocity), "Linear Bicycle Model with neglected fork angle (lambda=90deg, c=0) \"THE SIMPLEST MODEL\""/3(velocity), Linear Bicycle Model/3(velocity)
  Real Bike Parameters4/1 -> Linear Bicycle Model/6(parameters_f_b_real)
  Demux/3 -> " Addition of oscillations"/3(Roll Rate)  "True Roll Rate"
  " Addition of oscillations"/1(True States) -> Demux2/1, True States/1
  Demux2/2 -> Global Angles and Coordinates Calculator - Position/2(True Steering Angle)  "True Steering Angle"
  Global Angles and Coordinates Calculator - Position/1(True Position) -> True Position/1, Path Plotter Reality/1(Position)

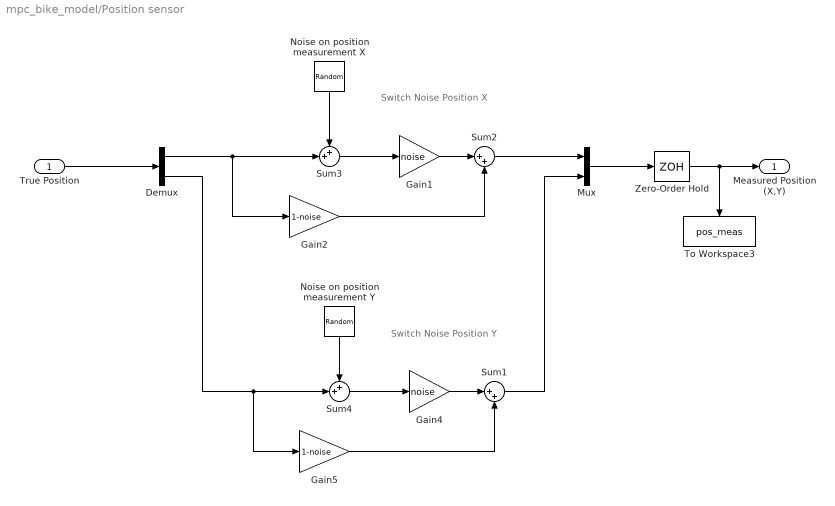
== system mpc_bike_model/Position sensor ==
  note: Switch Noise
      | Position X
  note: Switch Noise
      | Position Y
  True Position : Inport
  Demux : Demux  Outputs=2
  Gain1 : Gain  Gain=noise
  Gain2 : Gain  Gain=1-noise
  Gain4 : Gain  Gain=noise
  Gain5 : Gain  Gain=1-noise
  Mux : Mux  Inputs=2
  "Noise on position measurement X    " : RandomNumber  Variance=noise_pos_meas  Seed=2  SampleTime=Ts
  "Noise on position measurement Y     " : RandomNumber  Variance=noise_pos_meas  SampleTime=Ts
  Sum1 : Sum  Inputs=|++
  Sum2 : Sum  Inputs=|++
  Sum3 : Sum  Inputs=++|
  Sum4 : Sum  Inputs=++|
  To Workspace3 : ToWorkspace  VariableName=pos_meas  SaveFormat=Timeseries  SampleTime=-1
  Zero-Order Hold : ZeroOrderHold  SampleTime=Ts
  "Measured Position (X,Y) " : Outport
  wires:
  Zero-Order Hold/1 -> To Workspace3/1, "Measured Position (X,Y) "/1
  True Position/1 -> Demux/1
  Sum2/1 -> Mux/1
  Mux/1 -> Zero-Order Hold/1
  "Noise on position measurement X    "/1 -> Sum3/1
  Gain2/1 -> Sum2/2
  Demux/1 -> Gain2/1, Sum3/2
  "Noise on position measurement Y     "/1 -> Sum4/1
  Gain5/1 -> Sum1/2
  Demux/2 -> Sum4/2, Gain5/1
  Sum1/1 -> Mux/2
  Sum3/1 -> Gain1/1
  Gain1/1 -> Sum2/1
  Gain4/1 -> Sum1/1
  Sum4/1 -> Gain4/1

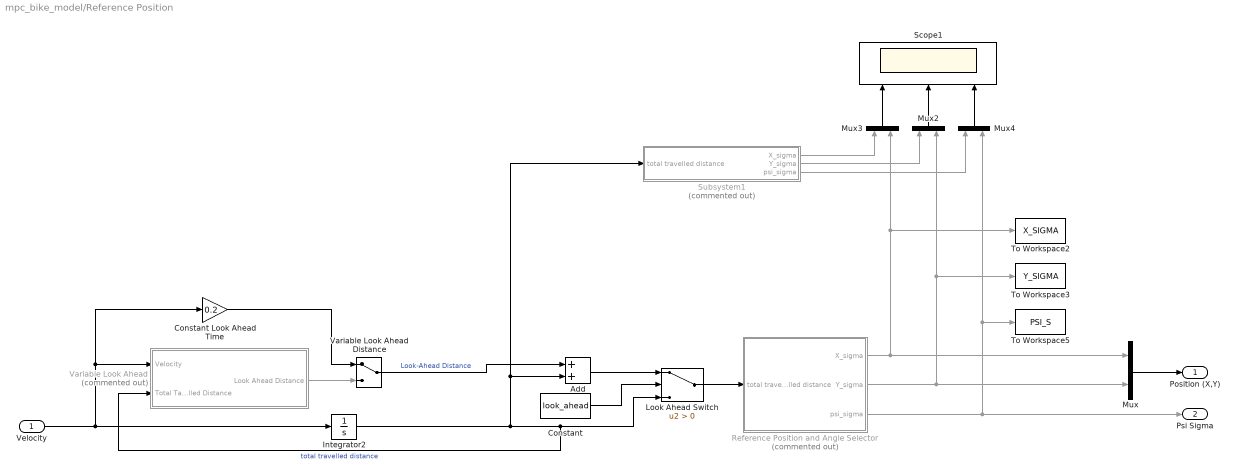
== system mpc_bike_model/Reference Position  ==
  Velocity : Inport
  Add : Sum
  Constant : Constant  Value=look_ahead
  Constant Look Ahead Time : Gain  Gain=0.2
  Integrator2 : Integrator
  Look Ahead Switch : Switch  Criteria=u2 > Threshold
  Mux{,2..4} (4 alike) : Mux  Inputs=2
  Reference Position and Angle Selector : Subsystem  Commented=on
  Scope1 : Scope  NumInputPorts=3
  Subsystem1 : Subsystem  Commented=on
  To Workspace2 : ToWorkspace  VariableName=X_SIGMA  SaveFormat=Timeseries  SampleTime=Ts
  To Workspace3 : ToWorkspace  VariableName=Y_SIGMA  SaveFormat=Timeseries  SampleTime=Ts
  To Workspace5 : ToWorkspace  VariableName=PSI_S  SaveFormat=Timeseries  SampleTime=Ts
  Variable Look Ahead Distance : ManualSwitch
  Variable Look Ahead : Subsystem  Commented=on
  Position (X,Y) : Outport
  Psi Sigma : Outport  Port=2
  wires:
  Constant Look Ahead Time/1 -> Variable Look Ahead Distance/1
  Reference Position and Angle Selector/3(psi_sigma) -> To Workspace5/1, Mux4/2, Psi Sigma/1
  Mux3/1 -> Scope1/1
  Subsystem1/3(psi_sigma) -> Mux4/1
  Mux2/1 -> Scope1/2
  Mux4/1 -> Scope1/3
  Velocity/1 -> Integrator2/1, Constant Look Ahead Time/1, Variable Look Ahead/1(Velocity)
  Add/1 -> Look Ahead Switch/1
  Reference Position and Angle Selector/2(Y_sigma) -> To Workspace3/1, Mux2/2, Mux/2
  Look Ahead Switch/1 -> Reference Position and Angle Selector/1(total travelled distance)
  Subsystem1/2(Y_sigma) -> Mux2/1
  Integrator2/1 -> Variable Look Ahead/2(Total Tavelled Distance), Look Ahead Switch/3, Subsystem1/1(total travelled distance), Add/2  "total travelled distance"
  Subsystem1/1(X_sigma) -> Mux3/1
  Reference Position and Angle Selector/1(X_sigma) -> Mux3/2, To Workspace2/1, Mux/1
  Variable Look Ahead Distance/1 -> Add/1  "Look-Ahead Distance"
  Constant/1 -> Look Ahead Switch/2
  Mux/1 -> Position (X,Y)/1
  Variable Look Ahead/1(Look Ahead Distance) -> Variable Look Ahead Distance/2

== system mpc_bike_model/Reference Velocity  ==
  note: If you will use this variable velocity
      | reference generator, you need to change
      | upper and lower limits of velocity specified
      | in initialization code!
  Add : Sum  Inputs=4
  Constant Velocity : Constant  Value=input_velocity
  Ramp : simulink/Sources/Ramp  slope=0.03  start=0  InitialOutput=0
  Reference Velocity Selector : ManualSwitch
  Sine Wave : Sin  Amplitude=0  SampleTime=0
  Step : Step  Time=20  Before=4  After=8  SampleTime=0
  Step1 : Step  Time=40  After=-1  SampleTime=0
  Reference Velocity : Outport
  wires:
  Ramp/1 -> Add/4
  Constant Velocity/1 -> Reference Velocity Selector/1
  Step1/1 -> Add/3
  Step/1 -> Add/2
  Sine Wave/1 -> Add/1
  Add/1 -> Reference Velocity Selector/2
  Reference Velocity Selector/1 -> Reference Velocity/1

== system mpc_bike_model/Steering Encoder ==
  note: Switch Noise
  note: True Steering
      | Angle
  True Steering Angle : Inport
  Demux : Demux  Outputs=3
  Gain1 : Gain  Gain=noise
  Gain2 : Gain  Gain=1-noise
  Noise on steering encoder : RandomNumber  Variance=noise_encoder  Seed=6  SampleTime=Ts
  Sum : Sum  Inputs=++|
  Sum1 : Sum  Inputs=|++
  Zero-Order Hold : ZeroOrderHold  SampleTime=Ts
  Measured Steering Angle : Outport
  wires:
  Sum/1 -> Gain1/1
  Sum1/1 -> Zero-Order Hold/1
  Zero-Order Hold/1 -> Measured Steering Angle/1
  Noise on steering encoder/1 -> Sum/1
  True Steering Angle/1 -> Demux/1
  Demux/2 -> Gain2/1, Sum/2
  Gain2/1 -> Sum1/2
  Gain1/1 -> Sum1/1

== system mpc_bike_model/Steering Motor ==
  Reference Steering Rate : Inport
  Measured States : Inport  Port=2
  Constant : Constant  Value=steering_motor_limitations
  Motor Delay : TransportDelay  DelayTime=delay
  Motor Deadband : Subsystem
  Rate Limiter : RateLimiter  RisingSlewLimit=max_steering_motor_acc  FallingSlewLimit=min_steering_motor_acc  SampleTimeMode=inherited
  Saturation : Saturate  UpperLimit=max_steering_motor_speed  LowerLimit=min_steering_motor_speed
  Switch : Switch  Criteria=u2 > Threshold
  To Workspace : ToWorkspace  VariableName=calculated_input  SaveFormat=Timeseries  SampleTime=Ts
  To Workspace1 : ToWorkspace  VariableName=realised_input  SaveFormat=Timeseries  SampleTime=Ts
  Velocity Saturation wrt Max and Min Handle Bar Angles : Subsystem
  Zero-Order Hold2 : ZeroOrderHold  SampleTime=Ts
  Output Steering Rate : Outport
  wires:
  Measured States/1 -> Velocity Saturation wrt Max and Min Handle Bar Angles/2(States)
  Motor Delay/1 -> Rate Limiter/1
  Constant/1 -> Switch/2
  Switch/1 -> Velocity Saturation wrt Max and Min Handle Bar Angles/1(Reference Steering Rate)
  Rate Limiter/1 -> Saturation/1
  Saturation/1 -> Switch/1
  Velocity Saturation wrt Max and Min Handle Bar Angles/1(Output Steering Rate) -> Zero-Order Hold2/1
  Motor Deadband/1(Input Signal After Dead Band) -> Motor Delay/1
  Zero-Order Hold2/1 -> Output Steering Rate/1, To Workspace1/1
  Reference Steering Rate/1 -> Switch/3, To Workspace/1, Motor Deadband/1(Calculated Input)

== system mpc_bike_model/Balance Controller/LQR Controller ==
  note: Input = steering angular velocity
  Velocity : Inport
  State Error : Inport  Port=2
  1-D Lookup Table : Lookup_n-D  NumberOfTableDimensions=1  BreakpointsForDimension1=velocity_lqr  BreakpointsForDimension2=velocity_lqr  BreakpointsForDimension3=velocity_lqr  BreakpointsForDimension4=velocity_lqr  Table=lqr_gains(:,1)  InternalRulePriority=Speed  RndMeth=Simplest  InputSameDT=on
  1-D Lookup Table1 : Lookup_n-D  NumberOfTableDimensions=1  BreakpointsForDimension1=velocity_lqr  BreakpointsForDimension2=velocity_lqr  BreakpointsForDimension3=velocity_lqr  BreakpointsForDimension4=velocity_lqr  Table=lqr_gains(:,2)  InternalRulePriority=Speed  RndMeth=Simplest  InputSameDT=on
  1-D Lookup Table2 : Lookup_n-D  NumberOfTableDimensions=1  BreakpointsForDimension1=velocity_lqr  BreakpointsForDimension2=velocity_lqr  BreakpointsForDimension3=velocity_lqr  BreakpointsForDimension4=velocity_lqr  Table=lqr_gains(:,3)  InternalRulePriority=Speed  RndMeth=Simplest  InputSameDT=on
  Display1 : Display
  Mux : Mux  Inputs=3
  Product : Product  Multiplication=Matrix(*)
  Scope : Scope
  Transpose : Math  Operator=transpose  SaturateOnIntegerOverflow=on
  Zero-Order Hold : ZeroOrderHold  SampleTime=Ts
  Zero-Order Hold1 : ZeroOrderHold  SampleTime=Ts
  Calculated Input : Outport
  wires:
  1-D Lookup Table/1 -> Mux/1  "K1"
  1-D Lookup Table1/1 -> Mux/2  "K2"
  State Error/1 -> Zero-Order Hold1/1
  Product/1 -> Zero-Order Hold/1
  1-D Lookup Table2/1 -> Mux/3  "K3"
  Velocity/1 -> 1-D Lookup Table2/1, 1-D Lookup Table1/1, 1-D Lookup Table/1
  Mux/1 -> Product/2, Display1/1
  Transpose/1 -> Product/1
  Zero-Order Hold/1 -> Calculated Input/1
  Zero-Order Hold1/1 -> Scope/1, Transpose/1

== system mpc_bike_model/Balance Controller/Reference States ==
  Velocity : Inport
  Delta Ref : Inport  Port=2
  Bike Parameters : Constant  Value=parameters_real
  Constant : Constant  Value=path_tracking
  Mux5 : Mux  Inputs=3
  Reference Roll Angle Calculator : MATLAB Function  TreatAsAtomicUnit=on
  Switch : Switch  Criteria=u2 > Threshold
  Reference States : Outport
  wires:
  Bike Parameters/1 -> Reference Roll Angle Calculator/1(parameters_real)
  Switch/1 -> Mux5/2, Reference Roll Angle Calculator/3(delta_ref)
  Reference Roll Angle Calculator/1(phi_ref) -> Mux5/1
  Velocity/1 -> Reference Roll Angle Calculator/2(velocity)
  Mux5/1 -> Reference States/1
  Constant/1 -> Switch/2
  Delta Ref/1 -> Switch/1

== system mpc_bike_model/Complementary filter/Complementary Filter ==
  Roll Angle Estimation due to Accelerometer : Inport
  Roll Rate due to Gyroscope : Inport  Port=2
  Delay : Delay  DelayLength=1  InitialCondition=initial_states(1)
  Gain2 : Gain  Gain=complementary
  Gain3 : Gain  Gain=1-complementary
  Gain4 : Gain  Gain=Ts_IMU
  Sum3 : Sum  Inputs=|++
  Sum4 : Sum  Inputs=++|
  Roll Angle Estimation : Outport
  wires:
  Roll Angle Estimation due to Accelerometer/1 -> Gain3/1  "Roll_acc"
  Sum3/1 -> Gain2/1
  Roll Rate due to Gyroscope/1 -> Gain4/1
  Delay/1 -> Sum3/2
  Gain4/1 -> Sum3/1
  Gain2/1 -> Sum4/2
  Gain3/1 -> Sum4/1
  Sum4/1 -> Delay/1, Roll Angle Estimation/1
